simulink model "task4_lqg"  (R2021b)
settings: Solver=FixedStepAuto  StartTime=0.0  StopTime=1000  FixedStep=0.005  RelTol=1e-3
undefined symbols (not defined in the file): A, B, C, D, K, L, Q1, R1, x0, x0obs
settings Model: Creator=den  LastModifiedBy=den

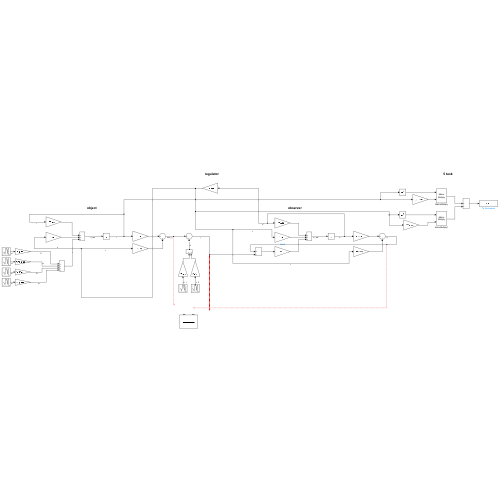
[thumbnail: Simulink's stored preview of the top-level diagram]
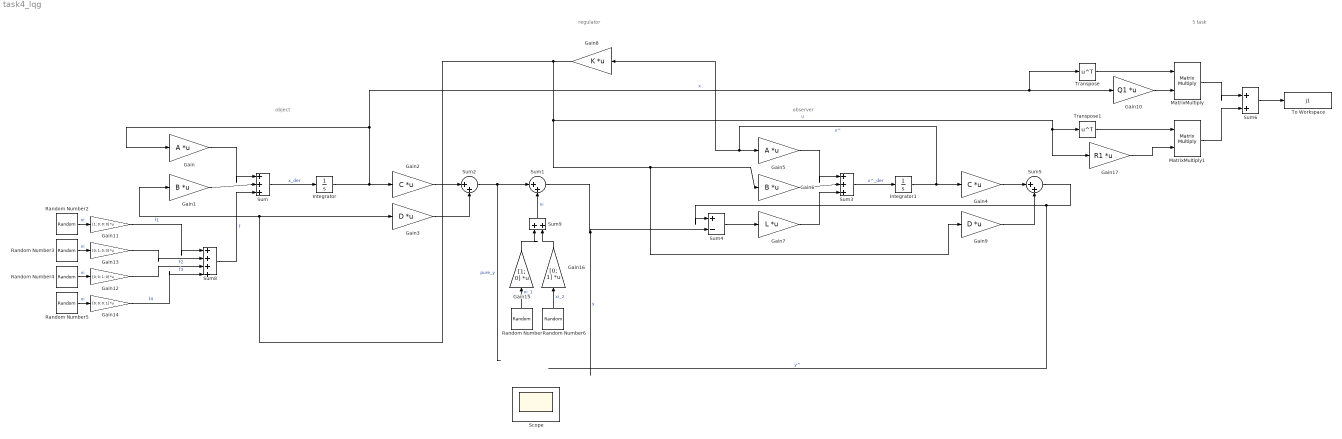
== system task4_lqg ==
  note: object
  note: observer
  note: regulator
  note: 5 task
  Gain : Gain  Gain=A  Multiplication=Matrix(K*u) (u vector)
  Gain1 : Gain  Gain=B  Multiplication=Matrix(K*u) (u vector)
  Gain10 : Gain  Gain=Q1  Multiplication=Matrix(K*u) (u vector)
  Gain11 : Gain  Gain=[1; 0; 0; 0]  Multiplication=Matrix(K*u) (u vector)
  Gain12 : Gain  Gain=[0; 0; 1; 0]  Multiplication=Matrix(K*u) (u vector)
  Gain13 : Gain  Gain=[0; 1; 0; 0]  Multiplication=Matrix(K*u) (u vector)
  Gain14 : Gain  Gain=[0; 0; 0; 1]  Multiplication=Matrix(K*u) (u vector)
  Gain15 : Gain  Gain=[1; 0]  Multiplication=Matrix(K*u) (u vector)
  Gain16 : Gain  Gain=[0; 1]  Multiplication=Matrix(K*u) (u vector)
  Gain17 : Gain  Gain=R1  Multiplication=Matrix(K*u) (u vector)
  Gain2 : Gain  Gain=C  Multiplication=Matrix(K*u) (u vector)
  Gain3 : Gain  Gain=D  Multiplication=Matrix(K*u) (u vector)
  Gain4 : Gain  Gain=C  Multiplication=Matrix(K*u) (u vector)
  Gain5 : Gain  Gain=A  Multiplication=Matrix(K*u) (u vector)
  Gain6 : Gain  Gain=B  Multiplication=Matrix(K*u) (u vector)
  Gain7 : Gain  Gain=L  Multiplication=Matrix(K*u) (u vector)
  Gain8 : Gain  Gain=K  Multiplication=Matrix(K*u) (u vector)
  Gain9 : Gain  Gain=D  Multiplication=Matrix(K*u) (u vector)
  Integrator : Integrator  InitialCondition=x0
  Integrator1 : Integrator  InitialCondition=x0obs
  MatrixMultiply : Product  Multiplication=Matrix(*)
  MatrixMultiply1 : Product  Multiplication=Matrix(*)
  Random Number : RandomNumber  Variance=19  Seed=99999  SampleTime=0.005
  Random Number2 : RandomNumber  Variance=15  Seed=9  SampleTime=0.005  VectorParams1D=off
  Random Number3 : RandomNumber  Variance=9  Seed=99  SampleTime=0.005  VectorParams1D=off
  Random Number4 : RandomNumber  Variance=29  Seed=999  SampleTime=0.005  VectorParams1D=off
  Random Number5 : RandomNumber  Variance=33  Seed=9999  SampleTime=0.005  VectorParams1D=off
  Random Number6 : RandomNumber  Variance=5  Seed=999999  SampleTime=0.005
  Scope : Scope  NumInputPorts=2
  Sum : Sum  Inputs=|+++
  Sum{1..2,5..6,9} (5 alike) : Sum  Inputs=|++
  Sum3 : Sum  Inputs=|+++
  Sum4 : Sum  Inputs=|+-
  Sum8 : Sum  Inputs=|++++
  To Workspace : ToWorkspace  VariableName=j1  SaveFormat=Structure With Time  SampleTime=-1
  Transpose : Math  Operator=transpose  SaturateOnIntegerOverflow=on
  Transpose1 : Math  Operator=transpose  SaturateOnIntegerOverflow=on
  wires:
  Gain/1 -> Sum/1
  Gain1/1 -> Sum/2
  Random Number4/1 -> Gain12/1  "xi"
  Random Number3/1 -> Gain13/1  "xi"
  Random Number5/1 -> Gain14/1  "xi"
  Random Number2/1 -> Gain11/1  "xi"
  Gain11/1 -> Sum8/1  "f1"
  Gain13/1 -> Sum8/2  "f2"
  Gain12/1 -> Sum8/3  "f3"
  Gain14/1 -> Sum8/4  "f4"
  Sum8/1 -> Sum/3  "f"
  Sum/1 -> Integrator/1  "x_der"
  Integrator/1 -> Gain2/1, Transpose/1, Gain10/1, Gain/1  "x"
  Sum1/1 -> Sum4/2  "y"
  Gain16/1 -> Sum9/2
  Gain15/1 -> Sum9/1
  Random Number/1 -> Gain15/1  "xi_1"
  Random Number6/1 -> Gain16/1  "xi_2"
  Sum9/1 -> Sum1/2  "xi"
  Gain2/1 -> Sum2/1
  Sum2/1 -> Sum1/1  "pure_y"
  Gain3/1 -> Sum2/2
  Gain8/1 -> Gain17/1, Transpose1/1, Gain9/1, Gain6/1, Gain1/1, Gain3/1  "u"
  Gain5/1 -> Sum3/1
  Gain6/1 -> Sum3/2
  Gain7/1 -> Sum3/3
  Sum4/1 -> Gain7/1
  Integrator1/1 -> Gain4/1, Gain5/1, Gain8/1  "x^"
  Sum3/1 -> Integrator1/1  "x^_der"
  Gain4/1 -> Sum5/1
  Gain9/1 -> Sum5/2
  Sum5/1 -> Sum4/1  "y^"
  Transpose/1 -> MatrixMultiply/1
  Gain10/1 -> MatrixMultiply/2
  MatrixMultiply/1 -> Sum6/1
  MatrixMultiply1/1 -> Sum6/2
  Transpose1/1 -> MatrixMultiply1/1
  Gain17/1 -> MatrixMultiply1/2
  Sum6/1 -> To Workspace/1
